simulink model "SIMULINK_04_ADAPTITIVE_CONTROL"  (R2020a)
settings: Solver=FixedStepAuto  StartTime=0.0  StopTime=600  FixedStep=0.01  RelTol=0.1e-3
libraries: simulink x1
settings Model: Creator=elkin  LastModifiedBy=USUARIO
settings SolverCC: AlgebraicLoopSolver=LineSearch

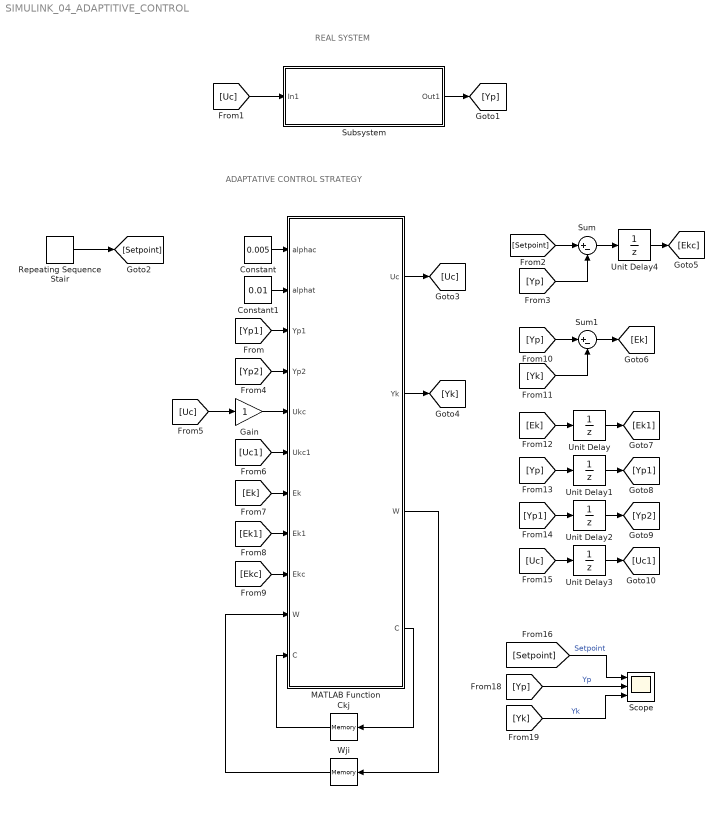
== system SIMULINK_04_ADAPTITIVE_CONTROL ==
  note: REAL SYSTEM
  note: ADAPTATIVE CONTROL STRATEGY
  Ckj : Memory  InitialCondition=rand(1,10)
  Constant : Constant  Value=0.005
  Constant1 : Constant  Value=0.01
  Gain : Gain
  MATLAB Function : MATLAB Function  TreatAsAtomicUnit=on
  Repeating Sequence Stair : simulink/Sources/Repeating Sequence Stair  OutValues=[0.4 0.2 0 0.4 0.8 0.4 1].'  tsamp=25  OutMin=[]  OutMax=[]  OutDataTypeStr=double  OutputDataTypeScalingMode=double  OutDataType=fixdt(0,8)  ConRadixGroup=Best Precision: Vector-wise  OutScaling=2^-12
  Scope : Scope  NumInputPorts=3
  Subsystem : Subsystem
  Sum : Sum  Inputs=|+-
  Sum1 : Sum  Inputs=|+-
  Unit Delay{,1..4} (5 alike) : UnitDelay  SampleTime=-1  HasFrameUpgradeWarning=on
  Wji : Memory  InitialCondition=rand(10,6)
  wires:
  Constant/1 -> MATLAB Function/1(alphac)
  Constant1/1 -> MATLAB Function/2(alphat)
  MATLAB Function/3(W) -> Wji/1
  MATLAB Function/4(C) -> Ckj/1
  Wji/1 -> MATLAB Function/10("W ")
  Ckj/1 -> MATLAB Function/11("C ")
  Subsystem/1(Out1) -> [Yp]
  Repeating Sequence Stair/1 -> [Setpoint]
  [Uc] -> Subsystem/1(In1)
  MATLAB Function/1(Uc) -> [Uc]
  MATLAB Function/2(Yk) -> [Yk]
  [Setpoint] -> Sum/1
  [Yp] -> Sum/2
  Sum/1 -> Unit Delay4/1
  [Yp1] -> MATLAB Function/3(Yp1)
  [Yp2] -> MATLAB Function/4(Yp2)
  [Ekc] -> MATLAB Function/9(Ekc)
  [Ek1] -> MATLAB Function/8(Ek1)
  [Ek] -> MATLAB Function/7(Ek)
  [Uc1] -> MATLAB Function/6(Ukc1)
  Gain/1 -> MATLAB Function/5(Ukc)
  [Uc] -> Gain/1
  [Yk] -> Sum1/2
  [Yp] -> Sum1/1
  Sum1/1 -> [Ek]
  [Ek] -> Unit Delay/1
  Unit Delay/1 -> [Ek1]
  Unit Delay1/1 -> [Yp1]
  [Yp] -> Unit Delay1/1
  Unit Delay2/1 -> [Yp2]
  [Yp1] -> Unit Delay2/1
  Unit Delay3/1 -> [Uc1]
  [Uc] -> Unit Delay3/1
  Unit Delay4/1 -> [Ekc]
  [Setpoint] -> Scope/1  "Setpoint"
  [Yk] -> Scope/3  "Yk"
  [Yp] -> Scope/2  "Yp"

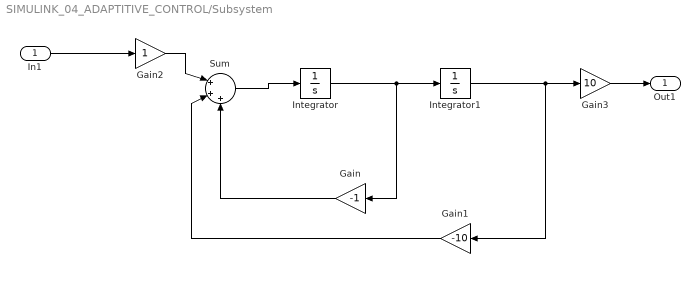
== system SIMULINK_04_ADAPTITIVE_CONTROL/Subsystem ==
  In1 : Inport
  Gain : Gain  Gain=-1
  Gain1 : Gain  Gain=-10
  Gain2 : Gain
  Gain3 : Gain  Gain=10
  Integrator : Integrator
  Integrator1 : Integrator
  Sum : Sum  Inputs=|+++
  Out1 : Outport  VectorParamsAs1DForOutWhenUnconnected=off
  wires:
  Integrator/1 -> Gain/1, Integrator1/1
  Gain2/1 -> Sum/1
  Gain1/1 -> Sum/2
  Sum/1 -> Integrator/1
  Integrator1/1 -> Gain3/1, Gain1/1
  Gain/1 -> Sum/3
  In1/1 -> Gain2/1
  Gain3/1 -> Out1/1

== matlab function SIMULINK_04_ADAPTITIVE_CONTROL/MATLAB Function ==
  data: alphac input; Uc output; Yk output; W output; C output; alphat input; Yp1 input; Yp2 input; Ukc input; Ukc1 input; Ek input; Ek1 input; Ekc input; W input; C input
% FUNCTION FOR ADAPTATIVE CONTROL STRUCTURE
% Santiago Garcia Arango
% ----------------------------------------------
% This functions develops a non-parametric identification and
% simultaneously creates a direct adaptative control strategy.

%    param alphat: The learning power of the non-parametric identification madaline neural network.
%    param alphac: The learning power of the adaptative controller.
%    param Yp1: First delay of the output of the system.
%    param Yp2: Second delay of the output of the system.
%    param Ukc: Current control signal.
%    param Ukc1: First delay of the control signal. 
%    param Ek: Current error signal of the non-parametric identification.
%    param Ek1: First delay of the error signal of the non-parametric identification.
%    param W: Neural weight matrix (First layer)
%    param C: Neural weight matrix (Second layer)
% -----------------------------------------------

function [Uc, Yk, W, C] = fcn(alphac, alphat, Yp1, Yp2, Ukc, Ukc1, Ek, Ek1, Ekc, W, C)
    % Define the inputs of the system
    inputs = [Yp1 Yp2 Ukc Ukc1 Ek Ek1];
    Xc = [0 0 1 0 0 0]; 
    
    % Calculate the output of the hidden layer
    Aj = W*inputs';
    H = tanh(Aj);
    
    % Calculate the output of the output layer
    Yk = C'*H;
    
    % Train of the neural network
    C = C + alphat*Ek*H;
    H2 = sech(Aj).^2; 
    W = W + alphat*Ek*(C.*H2)*inputs;
    
    % Calculate the control effort
    Uc = Ukc1 + alphac*Ekc*(C'*(W*Xc'));
